simulink model "testSim"  (R2024b)
settings: Solver=VariableStepAuto  StartTime=0.0  StopTime=t_final  RelTol=1e-3
values from neighbouring files (symbols this model uses):
  A = 0.2732    [analisi_teorica_cambio.m]
  crr_1 = 0.0013    [analisi_teorica_cambio.m]
  crr_2 = 0.000038    (= 3.8e-05)    [analisi_teorica_cambio.m]
  Cx_vec = [0.04179 0.03765 0.03503 0.03315 0.03172 0.03058 0.02981 0.02972 0.02972 0.02981 0.03010 0.03061 0.03133 0.03255 0.03397 0.03517 0.03648 0.03770]    [analisi_teorica_cambio.m]
  CxA_ref = 0.010344    [analisi_teorica_cambio.m]
  eta_tot = 0.97    [analisi_teorica_cambio.m]
  g = 9.81    [analisi_teorica_cambio.m]
  L = 2.63    [analisi_teorica_cambio.m]
  m = mv+mr+mw    (= 79)    [analisi_teorica_cambio.m]
  me = mr+mv+mw*1.5    (= 80.5)    [analisi_teorica_cambio.m]
  mu = 0.0000198    (= 1.98e-05)    [analisi_teorica_cambio.m]
  R_wheel = 0.23157    [analisi_teorica_cambio.m]
  rho = 0.97    [analisi_teorica_cambio.m]
  v_init = Vr(1)/3.6    [analisi_teorica_cambio.m]
  v_ref = 33.3333    [analisi_teorica_cambio.m]
  V_vec = [30:10:100 105:5:150]/3.6    [analisi_teorica_cambio.m]
libraries: simulink_extras x1
settings Model: Creator=mario  LastModifiedBy=mario

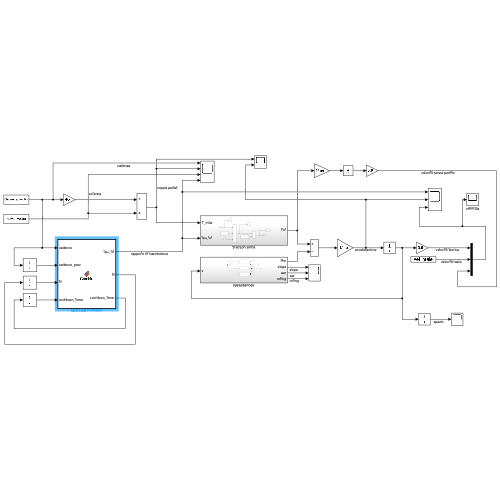
[thumbnail: Simulink's stored preview of the top-level diagram]
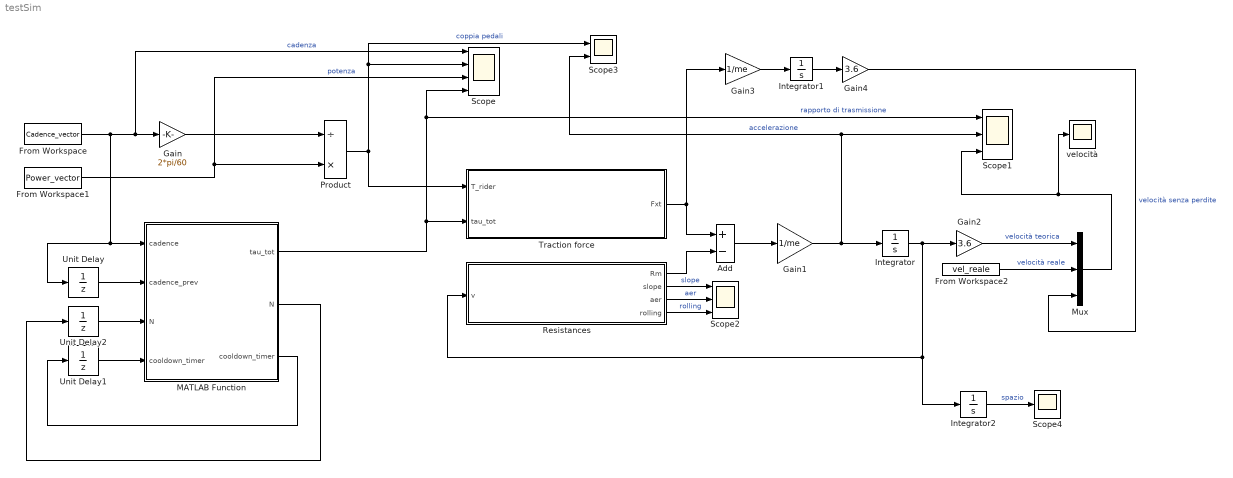
== system testSim ==
  Add : Sum  Inputs=+-
  From Workspace : FromWorkspace  VariableName=Cadence_vector
  From Workspace1 : FromWorkspace  VariableName=Power_vector
  From Workspace2 : FromWorkspace  VariableName=vel_reale
  Gain : Gain  Gain=2*pi/60
  Gain1 : Gain  Gain=1/me
  Gain2 : Gain  Gain=3.6
  Gain3 : Gain  Gain=1/me
  Gain4 : Gain  Gain=3.6
  Integrator : Integrator  InitialCondition=v_init
  Integrator1 : Integrator  InitialCondition=v_init
  Integrator2 : Integrator
  MATLAB Function : MATLAB Function  TreatAsAtomicUnit=on
  Mux : Mux  Inputs=3
  Product : Product  Inputs=/*
  Resistances : Subsystem
  Scope : Scope  NumInputPorts=4
  Scope1 : Scope  NumInputPorts=3
  Scope2 : Scope  NumInputPorts=3
  Scope3 : Scope  NumInputPorts=2
  Scope4 : Scope
  Traction force : Subsystem
  Unit Delay : UnitDelay  SampleTime=-1  HasFrameUpgradeWarning=on
  Unit Delay1 : UnitDelay  SampleTime=-1  HasFrameUpgradeWarning=on
  Unit Delay2 : UnitDelay  SampleTime=-1  HasFrameUpgradeWarning=on
  velocità : Scope
  wires:
  From Workspace/1 -> Gain/1, Scope/1, Unit Delay/1, MATLAB Function/1(cadence)  "cadenza"
  Gain/1 -> Product/1
  From Workspace1/1 -> Product/2, Scope/3  "potenza"
  Product/1 -> Traction force/1(T_rider), Scope/2, Scope3/1  "coppia pedali"
  Unit Delay/1 -> MATLAB Function/2(cadence_prev)
  Unit Delay1/1 -> MATLAB Function/4("cooldown_timer ")
  MATLAB Function/3(cooldown_timer) -> Unit Delay1/1
  Unit Delay2/1 -> MATLAB Function/3("N ")
  MATLAB Function/2(N) -> Unit Delay2/1
  MATLAB Function/1(tau_tot) -> Traction force/2(tau_tot), Scope/4, Scope1/1  "rapporto di trasmissione"
  Traction force/1(Fxt) -> Gain3/1, Add/1
  Resistances/1(Rm) -> Add/2
  Add/1 -> Gain1/1
  Gain1/1 -> Integrator/1, Scope3/2, Scope1/2  "accelerazione"
  Integrator/1 -> Gain2/1, Resistances/1(v), Integrator2/1
  Gain2/1 -> Mux/1  "velocità teorica"
  From Workspace2/1 -> Mux/2  "velocità reale"
  Mux/1 -> Scope1/3, velocità/1
  Resistances/2(slope) -> Scope2/1  "slope"
  Resistances/3(aer) -> Scope2/2  "aer"
  Resistances/4(rolling) -> Scope2/3  "rolling"
  Gain3/1 -> Integrator1/1
  Integrator1/1 -> Gain4/1
  Gain4/1 -> Mux/3  "velocità senza perdite"
  Integrator2/1 -> Scope4/1  "spazio"

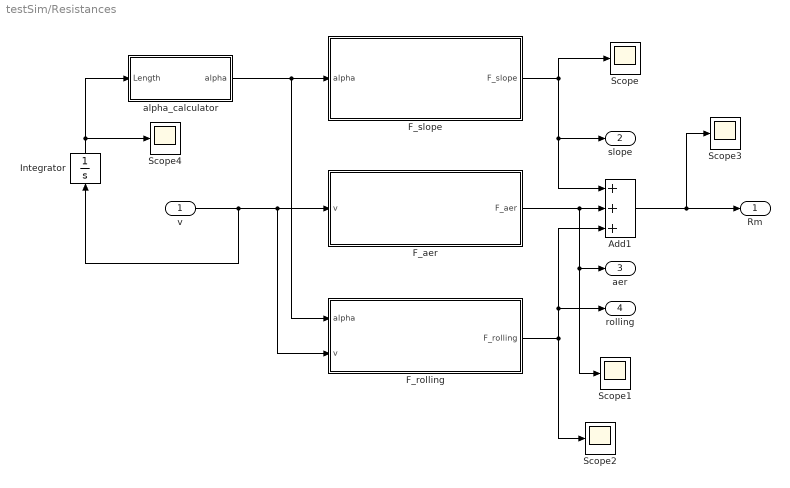
== system testSim/Resistances ==
  v : Inport
  Add1 : Sum  Inputs=+++
  F_aer : Subsystem
  F_rolling : Subsystem
  F_slope : Subsystem
  Integrator : Integrator
  Scope{,1..4} (5 alike) : Scope
  alpha_calculator : Subsystem
  Rm : Outport
  slope : Outport  Port=2
  aer : Outport  Port=3
  rolling : Outport  Port=4
  wires:
  F_slope/1(F_slope) -> slope/1, Add1/1, Scope/1
  v/1 -> Integrator/1, F_aer/1(v), F_rolling/2(v)
  Add1/1 -> Scope3/1, Rm/1
  F_rolling/1(F_rolling) -> Scope2/1, rolling/1, Add1/3
  F_aer/1(F_aer) -> aer/1, Scope1/1, Add1/2
  alpha_calculator/1(alpha) -> F_rolling/1(alpha), F_slope/1(alpha)
  Integrator/1 -> alpha_calculator/1(Length), Scope4/1

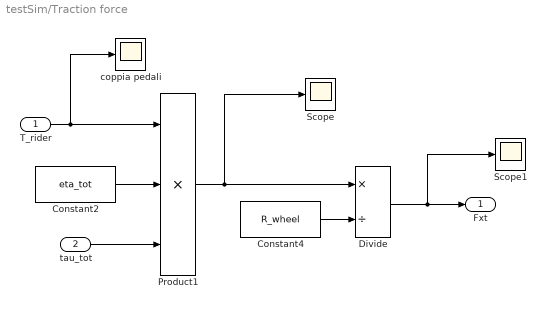
== system testSim/Traction force ==
  T_rider : Inport
  tau_tot : Inport  Port=2
  Constant2 : Constant  Value=eta_tot
  Constant4 : Constant  Value=R_wheel
  Divide : Product  Inputs=*/
  Product1 : Product  Inputs=3
  Scope : Scope
  Scope1 : Scope
  coppia pedali : Scope
  Fxt : Outport
  wires:
  T_rider/1 -> Product1/1, coppia pedali/1
  Constant4/1 -> Divide/2
  Product1/1 -> Divide/1, Scope/1
  Divide/1 -> Scope1/1, Fxt/1
  tau_tot/1 -> Product1/3
  Constant2/1 -> Product1/2

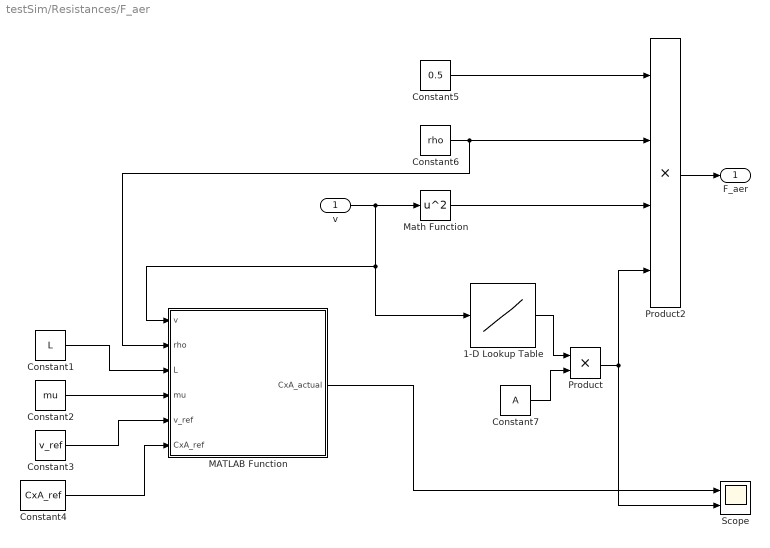
== system testSim/Resistances/F_aer ==
  v : Inport
  1-D Lookup Table : Lookup_n-D  NumberOfTableDimensions=1  BreakpointsForDimension1=V_vec  Table=Cx_vec  InternalRulePriority=Speed  RndMeth=Simplest
  Constant1 : Constant  Value=L
  Constant2 : Constant  Value=mu
  Constant3 : Constant  Value=v_ref
  Constant4 : Constant  Value=CxA_ref
  Constant5 : Constant  Value=0.5
  Constant6 : Constant  Value=rho
  Constant7 : Constant  Value=A
  MATLAB Function : MATLAB Function  TreatAsAtomicUnit=on
  Math Function : Math  Operator=square
  Product : Product
  Product2 : Product  Inputs=4
  Scope : Scope  NumInputPorts=2
  F_aer : Outport
  wires:
  Constant6/1 -> MATLAB Function/2(rho), Product2/2
  Constant5/1 -> Product2/1
  MATLAB Function/1(CxA_actual) -> Scope/1
  Product2/1 -> F_aer/1
  Math Function/1 -> Product2/3
  v/1 -> 1-D Lookup Table/1, MATLAB Function/1(v), Math Function/1
  Constant1/1 -> MATLAB Function/3(L)
  Constant2/1 -> MATLAB Function/4(mu)
  Constant3/1 -> MATLAB Function/5(v_ref)
  Constant4/1 -> MATLAB Function/6(CxA_ref)
  1-D Lookup Table/1 -> Product/1
  Constant7/1 -> Product/2
  Product/1 -> Scope/2, Product2/4

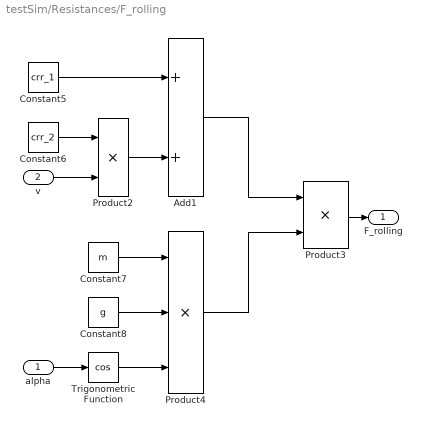
== system testSim/Resistances/F_rolling ==
  alpha : Inport
  v : Inport  Port=2
  Add1 : Sum
  Constant5 : Constant  Value=crr_1
  Constant6 : Constant  Value=crr_2
  Constant7 : Constant  Value=m
  Constant8 : Constant  Value=g
  Product2 : Product
  Product3 : Product
  Product4 : Product  Inputs=3
  Trigonometric Function : Trigonometry  Operator=cos
  F_rolling : Outport
  wires:
  Constant5/1 -> Add1/1
  Product3/1 -> F_rolling/1
  Constant6/1 -> Product2/1
  v/1 -> Product2/2
  Product2/1 -> Add1/2
  Trigonometric Function/1 -> Product4/3
  Constant7/1 -> Product4/1
  Constant8/1 -> Product4/2
  Product4/1 -> Product3/2
  alpha/1 -> Trigonometric Function/1
  Add1/1 -> Product3/1

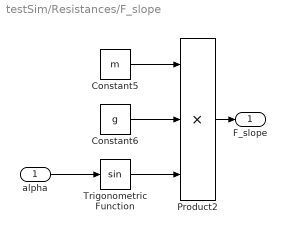
== system testSim/Resistances/F_slope ==
  alpha : Inport
  Constant5 : Constant  Value=m
  Constant6 : Constant  Value=g
  Product2 : Product  Inputs=3
  Trigonometric Function : Trigonometry
  F_slope : Outport
  wires:
  Constant6/1 -> Product2/2
  Product2/1 -> F_slope/1
  Constant5/1 -> Product2/1
  Trigonometric Function/1 -> Product2/3
  alpha/1 -> Trigonometric Function/1

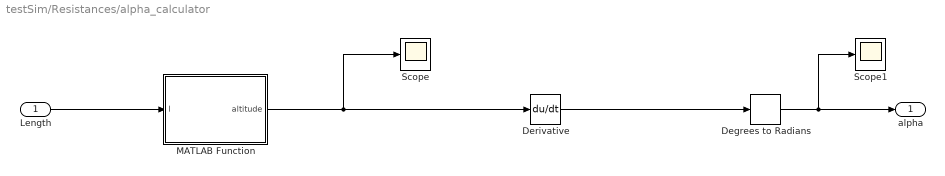
== system testSim/Resistances/alpha_calculator ==
  Length : Inport
  Degrees to Radians : simulink_extras/Transformations/Degrees to Radians
  Derivative : Derivative
  MATLAB Function : MATLAB Function  TreatAsAtomicUnit=on
  Scope : Scope
  Scope1 : Scope
  alpha : Outport
  wires:
  Degrees to Radians/1 -> alpha/1, Scope1/1
  Length/1 -> MATLAB Function/1(l)
  MATLAB Function/1(altitude) -> Scope/1, Derivative/1
  Derivative/1 -> Degrees to Radians/1

== matlab function testSim/Resistances/F_aer/MATLAB Function ==
  data: v input; CxA_actual output; rho input; L input; mu input; v_ref input; CxA_ref input
function CxA_actual = fcn(v,rho,L,mu,v_ref,CxA_ref)

Re = v*rho*L/mu;
Vect = [0.074*(Re^-0.2),0.01];
Num = min(Vect);
Den = 0.074*((v_ref*rho*L/mu)^-0.2);

CxA_actual = CxA_ref*Num/Den;

== matlab function testSim/MATLAB Function ==
  data: cadence input; tau_tot output; cadence_prev input; N input; cooldown_timer input; N output; cooldown_timer output
function [tau_tot, N, cooldown_timer] = Cambio(cadence, cadence_prev, N, cooldown_timer)
    cooldown_time = 3;       % evita rilevazioni continue non avendo la conferma della velocità (3-10)
    cadence_drop_threshold = -1.5;  % variazione significativa di cadenza (rpm) (0,5-2)

    delta_cad = cadence - cadence_prev;

    if cooldown_timer == 0
        if delta_cad < cadence_drop_threshold
            N = min(N + 1, 12); 
            cooldown_timer = cooldown_time;  
        end
    else
        cooldown_timer = cooldown_timer - 1;
    end
    
    %% rapporti originali 
    % Selezione del rapporto T in base alla marcia N
    % switch N
    %     case 12, T = 12;
    %     case 11, T = 13;
    %     case 10, T = 14;
    %     case 9,  T = 15;
    %     case 8,  T = 17;
    %     case 7,  T = 19;
    %     case 6,  T = 21;
    %     case 5,  T = 24;
    %     case 4,  T = 27;
    %     case 3,  T = 31;
    %     case 2,  T = 35;
    %     case 1,  T = 40;
    %     otherwise, T = 40;
    % end


%% 7 raooprti, cooldown time = 1, cadence_drop_treshold = -0,5 vMax=120km/h
    % switch N
    %     case 7, T = 12;
    %     case 6, T = 14;
    %     case 5, T = 17;
    %     case 4, T = 21;
    %     case 3, T = 24;
    %     case 2, T = 31;
    %     case 1, T = 40;
    %     otherwise, T = 40;
    % end

 %% 5 raooprti, cooldown time = 5, cadence_drop_treshold = -1,5 vMax=138km/h
    % switch N
    %     case 5, T = 17;
    %     case 4, T = 21;
    %     case 3, T = 24;
    %     case 2, T = 31;
    %     case 1, T = 40;
    %     otherwise, T = 40;
    % end

%% 6 rapporti, cooldown time = 3, cadence_drop_treshold = -0,5 vMax = 164km/h di picco 
    switch N
        case 6, T = 14;
        case 5, T = 21;
        case 4, T = 31;
        case 3, T = 40;
        case 2, T = 45;
        case 1, T = 50;
        otherwise, T = 50;
    end

%%

    tau_tot = (T / 108) * (18 / 38);

== matlab function testSim/Resistances/alpha_calculator/MATLAB Function ==
  data: l input; altitude output
function altitude = fcn(l)

altitude = -5.93e-15*l^4+2.22e-10*l^3-2.349e-06*l^2+0.003799*l+31.33;

end
